simulink model "MAX938_lipflop"  (R2022b)
settings: Solver=VariableStepAuto  StartTime=0.0  StopTime=10.0  RelTol=1e-3
libraries: simulink_extras x2
settings Model: Creator=hruda  LastModifiedBy=hruda

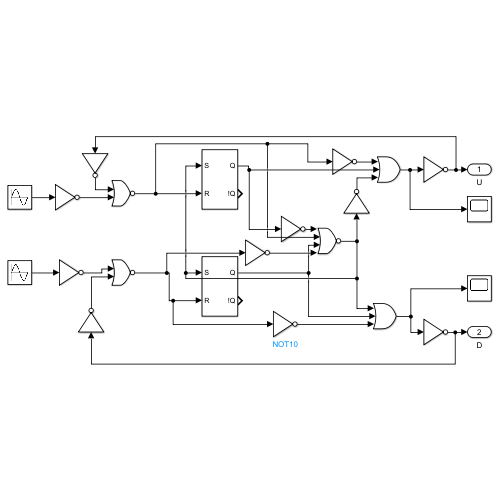
[thumbnail: Simulink's stored preview of the top-level diagram]
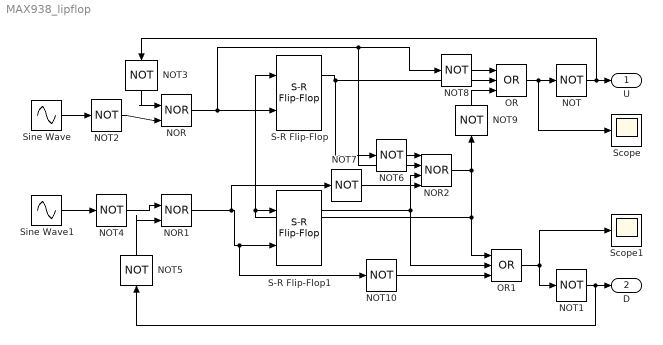
== system MAX938_lipflop ==
  NOR : Logic  Operator=NOR  IconShape=distinctive  AllPortsSameDT=off  OutDataTypeStr=boolean
  NOR1 : Logic  Operator=NOR  IconShape=distinctive  AllPortsSameDT=off  OutDataTypeStr=boolean
  NOR2 : Logic  Operator=NOR  Inputs=4  IconShape=distinctive  AllPortsSameDT=off  OutDataTypeStr=boolean
  NOT{,1..10} (11 alike) : Logic  Operator=NOT  IconShape=distinctive  AllPortsSameDT=off  OutDataTypeStr=boolean
  OR : Logic  Operator=OR  Inputs=3  IconShape=distinctive  AllPortsSameDT=off  OutDataTypeStr=boolean
  OR1 : Logic  Operator=OR  Inputs=3  IconShape=distinctive  AllPortsSameDT=off  OutDataTypeStr=boolean
  S-R Flip-Flop : simulink_extras/Flip Flops/S-R Flip-Flop  initial_condition=0
  S-R Flip-Flop1 : simulink_extras/Flip Flops/S-R Flip-Flop  initial_condition=0
  Scope : Scope
  Scope1 : Scope
  Sine Wave : Sin  SampleTime=0
  Sine Wave1 : Sin  SampleTime=0
  U : Outport
  D : Outport  Port=2
  wires:
  NOR1/1 -> NOT7/1, NOT10/1, S-R Flip-Flop1/2
  NOR/1 -> NOR2/2, NOT8/1, S-R Flip-Flop/2
  OR/1 -> Scope/1, NOT/1
  OR1/1 -> Scope1/1, NOT1/1
  NOT1/1 -> NOT5/1, D/1
  NOR2/1 -> NOT9/1, OR1/1, S-R Flip-Flop/1, S-R Flip-Flop1/1
  S-R Flip-Flop/1 -> NOT6/1, OR/2
  S-R Flip-Flop1/1 -> OR1/2, NOR2/3
  NOT/1 -> NOT3/1, U/1
  Sine Wave/1 -> NOT2/1
  Sine Wave1/1 -> NOT4/1
  NOT2/1 -> NOR/2
  NOT4/1 -> NOR1/1
  NOT3/1 -> NOR/1
  NOT5/1 -> NOR1/2
  NOT6/1 -> NOR2/1
  NOT7/1 -> NOR2/4
  NOT8/1 -> OR/1
  NOT9/1 -> OR/3
  NOT10/1 -> OR1/3
